simulink model "pwm_avg_pred_controlled_system"  (R2017a)
settings: Solver=VariableStepAuto  StartTime=0.0  StopTime=t_f  RelTol=1e-3
values from neighbouring files (symbols this model uses):
  A = double(subs(A_sym, symbs, vals))    [load_params.m]
  B = double(subs(B_sym, symbs, vals))    [load_params.m]
  C = double(subs(C_sym, symbs, vals))    [load_params.m]    (also in load_pwm_avg_pred_controller.m = sysd.c; load_pwm_pred_controller.m = sysd.c)
  Ctilde = double(subs(Ctilde_sym, symbs, vals))    [load_params.m]
  torque_ref = n_val*k_i_val*i_ref    [load_params.m]
  Ts_val = 1e-2    (= 0.01)    [load_params.m]    (also in load_pwm_controller.m = 0.1; ss_value.m = 0.011)
  Vcc_val = 12    [load_params.m]
  x0 = [0; 0]    [sim_controlled_system.m]
settings Model: Creator=brunolnetto  LastModifiedBy=brunolnetto
settings SolverCC: AlgebraicLoopSolver=LineSearch

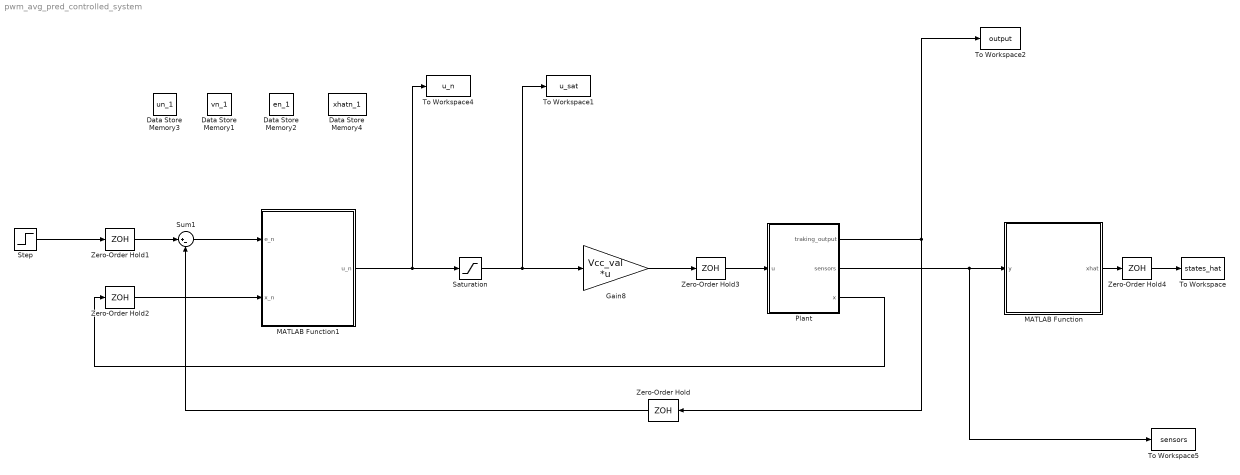
== system pwm_avg_pred_controlled_system ==
  Data Store Memory1 : DataStoreMemory  DataStoreName=vn_1  ReadBeforeWriteMsg=warning  WriteAfterWriteMsg=warning  WriteAfterReadMsg=warning  ShowAdditionalParam=off  OutDataTypeStr=double
  Data Store Memory2 : DataStoreMemory  DataStoreName=en_1  ReadBeforeWriteMsg=warning  WriteAfterWriteMsg=warning  WriteAfterReadMsg=warning  InitialValue=e0  ShowAdditionalParam=off  OutDataTypeStr=double
  Data Store Memory3 : DataStoreMemory  DataStoreName=un_1  ReadBeforeWriteMsg=warning  WriteAfterWriteMsg=warning  WriteAfterReadMsg=warning  ShowAdditionalParam=off  OutDataTypeStr=double
  Data Store Memory4 : DataStoreMemory  DataStoreName=xhatn_1  ReadBeforeWriteMsg=warning  WriteAfterWriteMsg=warning  WriteAfterReadMsg=warning  InitialValue=xhat0  ShowAdditionalParam=off  OutDataTypeStr=double
  Gain8 : Gain  Gain=Vcc_val  Multiplication=Matrix(K*u) (u vector)
  MATLAB Function : MATLAB Function  TreatAsAtomicUnit=on
  MATLAB Function1 : MATLAB Function  TreatAsAtomicUnit=on
  Plant : Subsystem
  Saturation : Saturate  UpperLimit=1  LowerLimit=-1
  Step : Step  Time=0  After=torque_ref  SampleTime=Ts_val
  Sum1 : Sum  Inputs=|+-
  To Workspace : ToWorkspace  VariableName=states_hat  SaveFormat=Structure With Time  SampleTime=-1
  To Workspace1 : ToWorkspace  VariableName=u_sat  SaveFormat=Structure With Time  SampleTime=-1
  To Workspace2 : ToWorkspace  VariableName=output  SaveFormat=Structure With Time  SampleTime=-1
  To Workspace4 : ToWorkspace  VariableName=u_n  SaveFormat=Structure With Time  SampleTime=-1
  To Workspace5 : ToWorkspace  VariableName=sensors  SaveFormat=Structure With Time  SampleTime=-1
  Zero-Order Hold{,1..4} (5 alike) : ZeroOrderHold  SampleTime=Ts_val
  wires:
  Zero-Order Hold1/1 -> Sum1/1
  Sum1/1 -> MATLAB Function1/1(e_n)
  MATLAB Function/1(xhat) -> Zero-Order Hold4/1
  Zero-Order Hold3/1 -> Plant/1(u)
  Step/1 -> Zero-Order Hold1/1
  Zero-Order Hold4/1 -> To Workspace/1
  Plant/3(x) -> Zero-Order Hold2/1
  Plant/1(traking_output) -> Zero-Order Hold/1, To Workspace2/1
  Zero-Order Hold/1 -> Sum1/2
  Zero-Order Hold2/1 -> MATLAB Function1/2(x_n)
  Plant/2(sensors) -> To Workspace5/1, MATLAB Function/1(y)
  Saturation/1 -> To Workspace1/1, Gain8/1
  MATLAB Function1/1(u_n) -> Saturation/1, To Workspace4/1
  Gain8/1 -> Zero-Order Hold3/1

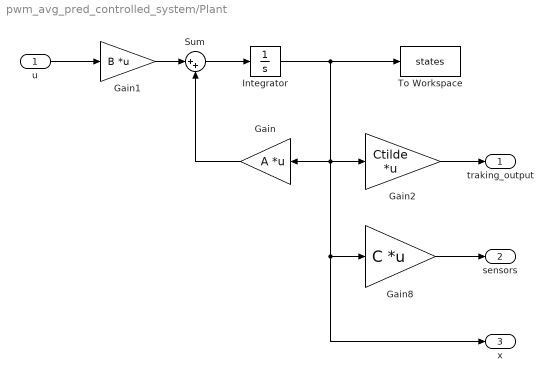
== system pwm_avg_pred_controlled_system/Plant ==
  u : Inport
  Gain : Gain  Gain=A  Multiplication=Matrix(K*u) (u vector)
  Gain1 : Gain  Gain=B  Multiplication=Matrix(K*u) (u vector)
  Gain2 : Gain  Gain=Ctilde  Multiplication=Matrix(K*u) (u vector)
  Gain8 : Gain  Gain=C  Multiplication=Matrix(K*u) (u vector)
  Integrator : Integrator  InitialCondition=x0
  Sum : Sum  Inputs=|++
  To Workspace : ToWorkspace  VariableName=states  SaveFormat=Structure With Time  SampleTime=-1
  traking_output : Outport
  sensors : Outport  Port=2
  x : Outport  Port=3
  wires:
  Gain8/1 -> sensors/1
  Gain1/1 -> Sum/1
  u/1 -> Gain1/1
  Gain/1 -> Sum/2
  Sum/1 -> Integrator/1
  Gain2/1 -> traking_output/1
  Integrator/1 -> To Workspace/1, Gain2/1, x/1, Gain8/1, Gain/1

== matlab function pwm_avg_pred_controlled_system/MATLAB Function ==
  data: y input; xhat output; un_1 data_store_memory; xhatn_1 data_store_memory; params parameter
function xhat = observador (y, params)
    global un_1;
    global xhatn_1;
    
    x_bar = params.Phi*xhatn_1 + params.Gamma*un_1;
    xhat = x_bar + params.L*(y - params.C*xhatn_1);

    xhatn_1 = xhat;
end

== matlab function pwm_avg_pred_controlled_system/MATLAB Function1 ==
  data: e_n input; x_n input; u_n output; vn_1 data_store_memory; params parameter; en_1 data_store_memory; un_1 data_store_memory
function u_n = controller(e_n, x_n, params)
    global vn_1;
    global en_1;
    global un_1;
    
    v_n = vn_1 + en_1;
    
    u_i = params.Ki*v_n;
    u_p = - params.Kp*x_n;
    
    u_n = u_i + u_p;
    
    vn_1 = v_n;
    en_1 = e_n;
    un_1 = u_n;
end
